simulink model "ecobot"  (R2014a)
settings: Solver=ode45  StartTime=0.0  StopTime=1000  RelTol=1e-3
values from neighbouring files (symbols this model uses):
  R = 4    [servo.m]
undefined symbols (not defined in the file or in its folder): d, Jt, km, n, r
libraries: simulink x1
settings Model: Creator=JinilGondalia  LastModifiedBy=JinilGondalia

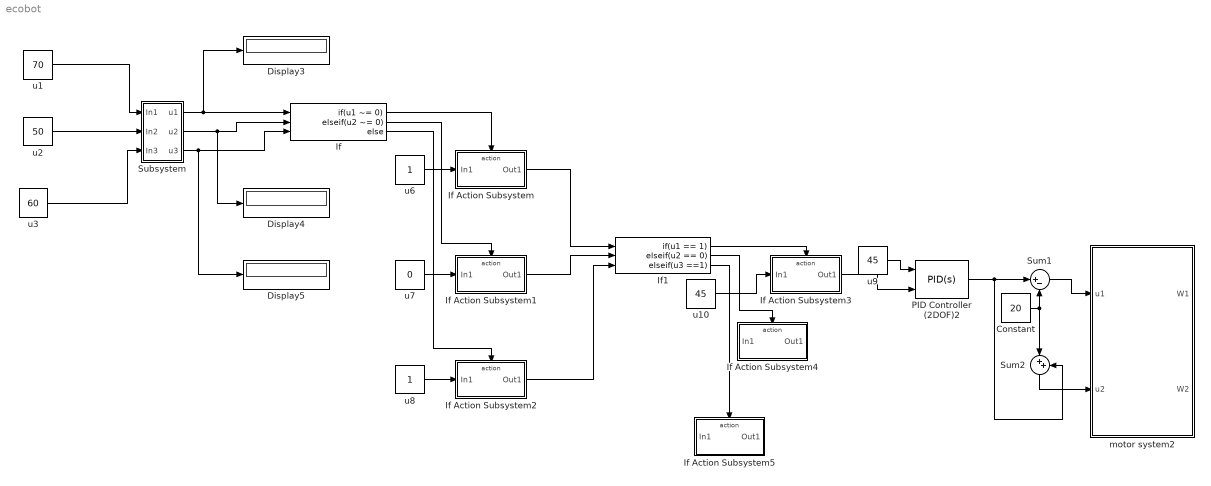
== system ecobot ==
  Constant : Constant  Value=20
  Display3 : Display
  Display4 : Display
  Display5 : Display
  If : If  NumInputs=3  IfExpression=u1 ~= 0  ElseIfExpressions=u2 ~= 0
  If Action Subsystem : Subsystem  TreatAsAtomicUnit=on
  If Action Subsystem1 : Subsystem  TreatAsAtomicUnit=on
  If Action Subsystem2 : Subsystem  TreatAsAtomicUnit=on
  If Action Subsystem3 : Subsystem  TreatAsAtomicUnit=on
  If Action Subsystem4 : Subsystem  TreatAsAtomicUnit=on
  If Action Subsystem5 : Subsystem  TreatAsAtomicUnit=on
  If1 : If  NumInputs=3  IfExpression=u1 == 1  ElseIfExpressions=u2 == 0, u3 ==1  ShowElse=off
  PID Controller (2DOF)2 : simulink/Continuous/PID Controller (2DOF)  Controller=PID  TimeDomain=Continuous-time  SampleTime=1  IntegratorMethod=Forward Euler  FilterMethod=Forward Euler  Form=Parallel  P=1  I=1  D=0  N=100  b=1  c=1  InitialConditionSource=internal  InitialConditionForIntegrator=0  InitialConditionForFilter=0  ExternalReset=none  LimitOutput=off  UpperSaturationLimit=10000  LowerSaturationLimit=-inf  LinearizeAsGain=on  AntiWindupMode=none  Kb=1  TrackingMode=off  Kt=1  PParamMin=[]  PParamMax=[]  IParamMin=[]  IParamMax=[]  DParamMin=[]  DParamMax=[]  NParamMin=[]  NParamMax=[]  bParamMin=[]  bParamMax=[]  cParamMin=[]  cParamMax=[]  KbParamMin=[]  KbParamMax=[]  KtParamMin=[]  KtParamMax=[]  POutMin=[]  POutMax=[]  IOutMin=[]  IOutMax=[]  DOutMin=[]  DOutMax=[]  NOutMin=[]  NOutMax=[]  bOutMin=[]  bOutMax=[]  cOutMin=[]  cOutMax=[]  KbOutMin=[]  KbOutMax=[]  KtOutMin=[]  KtOutMax=[]  IntegratorOutMin=[]  IntegratorOutMax=[]  FilterOutMin=[]  FilterOutMax=[]  SumOutMin=[]  SumOutMax=[]  Sum1OutMin=[]  Sum1OutMax=[]  Sum2OutMin=[]  Sum2OutMax=[]  Sum3OutMin=[]  Sum3OutMax=[]  SumI1OutMin=[]  SumI1OutMax=[]  SumI2OutMin=[]  SumI2OutMax=[]  SumI3OutMin=[]  SumI3OutMax=[]  SumDOutMin=[]  SumDOutMax=[]  SaturationOutMin=[]  SaturationOutMax=[]  IntegratorContinuousStateAttributes=''  IntegratorStateMustResolveToSignalObject=off  IntegratorRTWStateStorageClass=Auto  FilterContinuousStateAttributes=''  FilterStateMustResolveToSignalObject=off  FilterRTWStateStorageClass=Auto
  Subsystem : Subsystem
  Sum1 : Sum  Inputs=|+-
  Sum2 : Sum  Inputs=|++
  motor system2 : Subsystem
  u1 : Constant  Value=70
  u10 : Constant  Value=45
  u2 : Constant  Value=50
  u3 : Constant  Value=60
  u6 : Constant
  u7 : Constant  Value=0
  u8 : Constant
  u9 : Constant  Value=45
  wires:
  u1/1 -> Subsystem/1(In1)
  u2/1 -> Subsystem/2(In2)
  u3/1 -> Subsystem/3(In3)
  Subsystem/1("u1 ") -> Display3/1, If/1
  Subsystem/2(u2) -> Display4/1, If/2
  Subsystem/3(u3) -> Display5/1, If/3
  If/1 -> If Action Subsystem/Action
  u6/1 -> If Action Subsystem/1(In1)
  If/2 -> If Action Subsystem1/Action
  If/3 -> If Action Subsystem2/Action
  u8/1 -> If Action Subsystem2/1(In1)
  u7/1 -> If Action Subsystem1/1(In1)
  If Action Subsystem/1(Out1) -> If1/1
  If Action Subsystem1/1(Out1) -> If1/2
  If Action Subsystem2/1(Out1) -> If1/3
  If1/1 -> If Action Subsystem3/Action
  If1/2 -> If Action Subsystem4/Action
  If1/3 -> If Action Subsystem5/Action
  Constant/1 -> Sum2/1, Sum1/2
  If Action Subsystem3/1(Out1) -> PID Controller (2DOF)2/2
  Sum1/1 -> motor system2/1(u1)
  u9/1 -> PID Controller (2DOF)2/1
  u10/1 -> If Action Subsystem3/1(In1)
  PID Controller (2DOF)2/1 -> Sum2/2, Sum1/1
  Sum2/1 -> motor system2/2(u2)

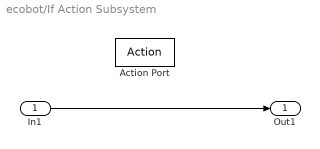
== system ecobot/If Action Subsystem ==
  In1 : Inport
  Action Port : ActionPort  ActionType=then
  Out1 : Outport
  wires:
  In1/1 -> Out1/1

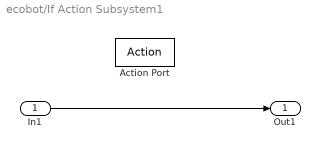
== system ecobot/If Action Subsystem1 ==
  In1 : Inport
  Action Port : ActionPort  ActionType=elseif
  Out1 : Outport
  wires:
  In1/1 -> Out1/1

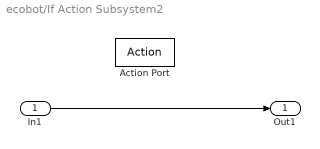
== system ecobot/If Action Subsystem2 ==
  In1 : Inport
  Action Port : ActionPort  ActionType=else
  Out1 : Outport
  wires:
  In1/1 -> Out1/1

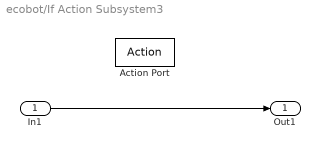
== system ecobot/If Action Subsystem3 ==
  In1 : Inport
  Action Port : ActionPort  ActionType=then
  Out1 : Outport
  wires:
  In1/1 -> Out1/1

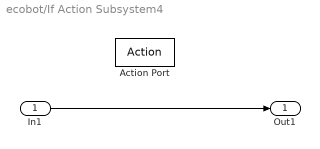
== system ecobot/If Action Subsystem4 ==
  In1 : Inport
  Action Port : ActionPort  ActionType=elseif
  Out1 : Outport
  wires:
  In1/1 -> Out1/1

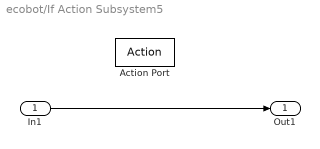
== system ecobot/If Action Subsystem5 ==
  In1 : Inport
  Action Port : ActionPort  ActionType=elseif
  Out1 : Outport
  wires:
  In1/1 -> Out1/1

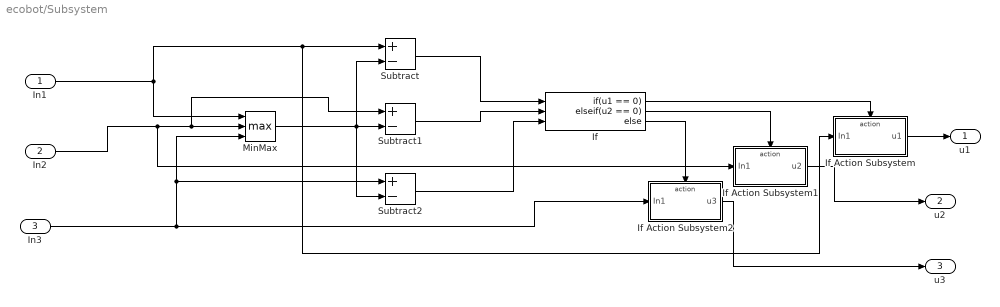
== system ecobot/Subsystem ==
  In1 : Inport
  In2 : Inport  Port=2
  In3 : Inport  Port=3
  If : If  NumInputs=3  IfExpression=u1 == 0  ElseIfExpressions=u2 == 0
  If Action Subsystem : Subsystem  TreatAsAtomicUnit=on
  If Action Subsystem1 : Subsystem  TreatAsAtomicUnit=on
  If Action Subsystem2 : Subsystem  TreatAsAtomicUnit=on
  MinMax : MinMax  Function=max  Inputs=3
  Subtract : Sum  Inputs=+-
  Subtract1 : Sum  Inputs=+-
  Subtract2 : Sum  Inputs=+-
  "u1 " : Outport
  u2 : Outport  Port=2
  u3 : Outport  Port=3
  wires:
  In3/1 -> If Action Subsystem2/1(In1), Subtract2/1, MinMax/3
  In1/1 -> If Action Subsystem/1(In1), Subtract/1, MinMax/1
  Subtract2/1 -> If/3
  In2/1 -> If Action Subsystem1/1(In1), Subtract1/1, MinMax/2
  If/2 -> If Action Subsystem1/Action
  MinMax/1 -> Subtract2/2, Subtract1/2, Subtract/2
  If/1 -> If Action Subsystem/Action
  If/3 -> If Action Subsystem2/Action
  Subtract1/1 -> If/2
  Subtract/1 -> If/1
  If Action Subsystem/1(u1) -> "u1 "/1
  If Action Subsystem1/1("u2 ") -> u2/1
  If Action Subsystem2/1(u3) -> u3/1

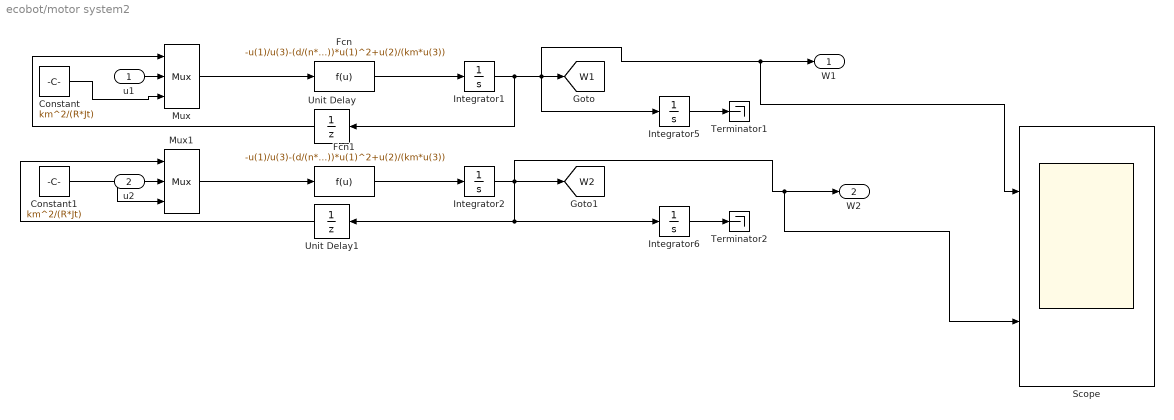
== system ecobot/motor system2 ==
  u1 : Inport
  u2 : Inport  Port=2
  Constant : Constant  Value=km^2/(R*Jt)
  Constant1 : Constant  Value=km^2/(R*Jt)
  Fcn : Fcn  Expr=-u(1)/u(3)-(d/(n*r^3*Jt))*u(1)^2+u(2)/(km*u(3))
  Fcn1 : Fcn  Expr=-u(1)/u(3)-(d/(n*r^3*Jt))*u(1)^2+u(2)/(km*u(3))
  Integrator{1..2,5..6} (4 alike) : Integrator
  Mux : Mux  Inputs=3
  Mux1 : Mux  Inputs=3
  Scope : Scope  NumInputPorts=2
      settings: YMin=-5~-5  YMax=5~5
  Terminator1 : Terminator
  Terminator2 : Terminator
  Unit Delay : UnitDelay  SampleTime=-1
  Unit Delay1 : UnitDelay  SampleTime=-1
  "W1 " : Outport
  W2 : Outport  Port=2
  tag scope: W1=global, W2=global
  wires:
  Unit Delay1/1 -> Mux1/1
  Unit Delay/1 -> Mux/1
  Integrator2/1 -> Unit Delay1/1, Integrator6/1, [W2], W2/1, Scope/2
  Integrator1/1 -> [W1], Integrator5/1, "W1 "/1, Scope/1, Unit Delay/1
  Integrator5/1 -> Terminator1/1
  Integrator6/1 -> Terminator2/1
  u2/1 -> Mux1/2
  Mux1/1 -> Fcn1/1
  Fcn1/1 -> Integrator2/1
  Constant1/1 -> Mux1/3
  u1/1 -> Mux/2
  Mux/1 -> Fcn/1
  Fcn/1 -> Integrator1/1
  Constant/1 -> Mux/3

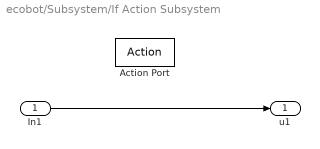
== system ecobot/Subsystem/If Action Subsystem ==
  In1 : Inport
  Action Port : ActionPort  ActionType=then
  u1 : Outport
  wires:
  In1/1 -> u1/1

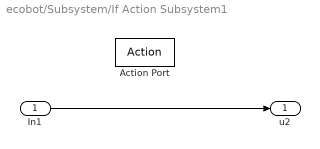
== system ecobot/Subsystem/If Action Subsystem1 ==
  In1 : Inport
  Action Port : ActionPort  ActionType=elseif
  "u2 " : Outport
  wires:
  In1/1 -> "u2 "/1

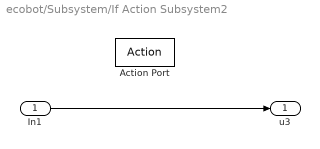
== system ecobot/Subsystem/If Action Subsystem2 ==
  In1 : Inport
  Action Port : ActionPort  ActionType=else
  u3 : Outport
  wires:
  In1/1 -> u3/1
